simulink model "SIL_swarm_Vasarhelyi"  (R2020b)
settings: Solver=FixedStepAuto  StartTime=0.0  StopTime=T  FixedStep=sim_rate  RelTol=1e-3  EnableMultiTasking=on
model workspace (MAT data in the model file):
  SL_ROS_VariableLengthArrays_MaxSizes : object (value not decoded)
undefined symbols (not defined in the file): airspeed_ref, Altitude_ref, DiscIntNeverNeededParam, Elevators, N_Waypoints, p_swarm, Propeller, Radius_waypoint, RightAileron, RightFlap, Rudder, Waypoints
libraries: robotlib x21, simulink x10, eeGeneralControl x5, dspvision x5
(part 2 of 4)

== system SIL_swarm_Vasarhelyi/Cessna 4/Controle de Direção ==
  Yaw : Inport
  X : Inport  Port=2
  Y : Inport  Port=3
  Y Ref : Inport  Port=4
  X Ref : Inport  Port=5
  Atan2 : Trigonometry  Operator=atan2
  Discrete Derivative : simulink/Discrete/Discrete Derivative  gainval=1.0  ICPrevScaledInput=0.0  OutMin=[]  OutMax=[]  OutDataType=fixdt(1, 16)  OutScaling=2^-10  DoSatur=off
  Discrete-Time Integrator : DiscreteIntegrator  SampleTime=-1  ICPrevOutput=DiscIntNeverNeededParam  ICPrevScaledInput=DiscIntNeverNeededParam
  Kd : Gain  Gain=3.0
  Ki : Gain  Gain=0.0
  Kp : Gain  Gain=1.6616
  Mux1 : Mux  Inputs=2
  Mux2 : Mux  Inputs=2
  Mux3 : Mux  Inputs=2
  Saturation : Saturate  UpperLimit=0.226893  LowerLimit=-0.226893
  Sum2 : Sum  Inputs=|+-
  Sum3 : Sum  Inputs=|+-
  Sum4 : Sum  Inputs=|+-
  Sum5 : Sum  Inputs=+++
  neg : Gain  Gain=-1
  yaw_error : Outport
  Roll Ref : Outport  Port=2
  guidance_error : Outport  Port=3
  wires:
  Mux1/1 -> Mux3/1
  Mux2/1 -> Mux3/2
  Saturation/1 -> neg/1
  neg/1 -> Roll Ref/1
  Sum3/1 -> Atan2/1
  Y/1 -> Sum3/2, Mux2/2
  Y Ref/1 -> Sum3/1, Mux2/1
  X Ref/1 -> Sum2/1, Mux1/1
  X/1 -> Sum2/2, Mux1/2
  Sum2/1 -> Atan2/2
  Atan2/1 -> Sum4/1
  Yaw/1 -> Sum4/2
  Mux3/1 -> guidance_error/1
  Sum5/1 -> Saturation/1
  Kp/1 -> Sum5/2
  Kd/1 -> Sum5/1
  Discrete Derivative/1 -> Kd/1
  Discrete-Time Integrator/1 -> Ki/1
  Sum4/1 -> Discrete-Time Integrator/1, Kp/1, Discrete Derivative/1, yaw_error/1
  Ki/1 -> Sum5/3

== system SIL_swarm_Vasarhelyi/Cessna 4/High-Level ==
  Pos : Inport
  Altitude ref : Inport  Port=2
  Xi : Inport  Port=3
  Bus Selector2 : BusSelector  OutputSignals=X,Y,Altitude
  Filtered Derivative Discrete : eeGeneralControl/Filtered Derivative (Discrete or Continuous)  K=1  T=0.001  B=inf  A=-inf  minRatio=10  init_option=Inherited from block input  x0=0  Ts=-1
      settings: SourceProductBaseCode=PS
  Gerador de Waypoints : Subsystem
  Mux : Mux  Inputs=3
  Mux1 : Mux  Inputs=3
  Terminator2 : Terminator
  Vasarhelyi Algorithm : Subsystem
  Velocity Direction : MATLAB Function  TreatAsAtomicUnit=on
  Y Ref : Outport
  X Ref : Outport  Port=2
  vel : Outport  Port=3
  u_ref : Outport  Port=4
  Waypoints : Outport  Port=5
  wires:
  Mux1/1 -> Waypoints/1, Velocity Direction/2(wp)
  Velocity Direction/1(u_ref) -> u_ref/1, Vasarhelyi Algorithm/3(u_ref)
  Pos/1 -> Bus Selector2/1
  Altitude ref/1 -> Mux1/3
  Gerador de Waypoints/2(Y Ref) -> Mux1/2
  Gerador de Waypoints/1(X Ref) -> Mux1/1
  Bus Selector2/1 -> Mux/1  "<X>"
  Bus Selector2/2 -> Mux/2  "<Y>"
  Bus Selector2/3 -> Mux/3  "<Altitude>"
  Mux/1 -> Filtered Derivative Discrete/1, Vasarhelyi Algorithm/1(pos_i), Velocity Direction/1(pos)
  Filtered Derivative Discrete/1 -> vel/1
  Xi/1 -> Vasarhelyi Algorithm/2(pqj)
  Vasarhelyi Algorithm/1(X) -> X Ref/1
  Vasarhelyi Algorithm/2(Y) -> Y Ref/1
  Vasarhelyi Algorithm/3(Z) -> Terminator2/1
  Vasarhelyi Algorithm/4(Xi) -> Gerador de Waypoints/1(Xi)

== system SIL_swarm_Vasarhelyi/Cessna 4/ROS Communication ==
  Profundor : Inport
  Rudder : Inport  Port=2
  Aileron : Inport  Port=3
  Throttle : Inport  Port=4
  Constant : Constant  Value=0
  Constant1 : Constant  Value=0
  Envio e Recepção de Dados do ROS : Subsystem
  Terminator2 : Terminator
  Roll : Outport
  Pitch : Outport  Port=2
  Yaw : Outport  Port=3
  ECEF Y : Outport  Port=4
  ECEF X : Outport  Port=5
  ECEF Z : Outport  Port=6
  Velocity : Outport  Port=7
  Xi : Outport  Port=8
  wires:
  Profundor/1 -> Envio e Recepção de Dados do ROS/2(Elevators)
  Constant/1 -> Envio e Recepção de Dados do ROS/3(Flap)
  Aileron/1 -> Envio e Recepção de Dados do ROS/4(Aileron)
  Envio e Recepção de Dados do ROS/1(Pitch) -> Pitch/1
  Envio e Recepção de Dados do ROS/4(ECEF X) -> ECEF X/1
  Envio e Recepção de Dados do ROS/5(ECEF Y) -> ECEF Y/1
  Envio e Recepção de Dados do ROS/2(Yaw) -> Yaw/1
  Envio e Recepção de Dados do ROS/3(Roll) -> Roll/1
  Envio e Recepção de Dados do ROS/6(ECEF Z) -> ECEF Z/1
  Envio e Recepção de Dados do ROS/7(Velocity) -> Velocity/1
  Rudder/1 -> Terminator2/1
  Envio e Recepção de Dados do ROS/8(Xi) -> Xi/1
  Throttle/1 -> Envio e Recepção de Dados do ROS/5(Propeller)
  Constant1/1 -> Envio e Recepção de Dados do ROS/1(Rudder)

== system SIL_swarm_Vasarhelyi/Cessna 5/Attitude Control ==
  note: bota po
  Vel ref : Inport
  Euler Angles : Inport  Port=2
  Roll_ref : Inport  Port=3
  Altitude : Inport  Port=4
  Vel_in : Inport  Port=5
  Altitude ref : Inport  Port=6
  Bus Selector : BusSelector  OutputSignals=Pitch,Roll,Yaw
  Constant : Constant  Value=0
  Controle de Altitude : Subsystem
  Controle de Velocidade : Subsystem
  Gain : Gain  Gain=-1
  Servo : Subsystem
  Sum1 : Sum  Inputs=|+-
  Sum3 : Sum  Inputs=+-|
  Sum5 : Sum  Inputs=+-|
  Z Take-off Ref : Constant  Value=5
  Profundor : Outport
  Rudder : Outport  Port=2
  Aileron : Outport  Port=3
  Throtlle : Outport  Port=4
  altitude_e : Outport  Port=5
  velocity_e : Outport  Port=6
  roll_e : Outport  Port=7
  wires:
  Roll_ref/1 -> Sum1/1  "Roll Ref"
  Constant/1 -> Sum5/1  "Yaw Ref"
  Servo/4(Throtlle) -> Throtlle/1
  Servo/2(Aileron) -> Aileron/1
  Servo/3(Rudder) -> Rudder/1
  Servo/1(Profundor) -> Profundor/1
  Z Take-off Ref/1 -> Servo/6(Altitude Ref)
  Altitude/1 -> Controle de Altitude/2(Altitude), Servo/5(Altitude)
  Gain/1 -> Sum3/2
  Sum5/1 -> Servo/3(Yaw Attitude)
  Bus Selector/3 -> Sum5/2  "<Yaw>"
  Sum3/1 -> Servo/1(Pitch Attitude)
  Euler Angles/1 -> Bus Selector/1
  Bus Selector/1 -> Gain/1  "<Pitch>"
  Bus Selector/2 -> Sum1/2  "<Roll>"
  Controle de Velocidade/1(Propeller Target) -> Servo/4(Vel_in)
  Controle de Altitude/1(Pitch_ref) -> Sum3/1
  Vel ref/1 -> Controle de Velocidade/1(Velocity Ref)
  Altitude ref/1 -> Controle de Altitude/1(Altitude Ref)
  Sum1/1 -> roll_e/1, Servo/2(Roll Attitude)
  Vel_in/1 -> Controle de Velocidade/2(Velocity)
  Controle de Altitude/2(altitude_error) -> altitude_e/1
  Controle de Velocidade/2(velocity_error) -> velocity_e/1

== system SIL_swarm_Vasarhelyi/Cessna 5/Controle de Direção ==
  Yaw : Inport
  X : Inport  Port=2
  Y : Inport  Port=3
  Y Ref : Inport  Port=4
  X Ref : Inport  Port=5
  Atan2 : Trigonometry  Operator=atan2
  Discrete Derivative : simulink/Discrete/Discrete Derivative  gainval=1.0  ICPrevScaledInput=0.0  OutMin=[]  OutMax=[]  OutDataType=fixdt(1, 16)  OutScaling=2^-10  DoSatur=off
  Discrete-Time Integrator : DiscreteIntegrator  SampleTime=-1  ICPrevOutput=DiscIntNeverNeededParam  ICPrevScaledInput=DiscIntNeverNeededParam
  Kd : Gain  Gain=3.0
  Ki : Gain  Gain=0.0
  Kp : Gain  Gain=1.6616
  Mux1 : Mux  Inputs=2
  Mux2 : Mux  Inputs=2
  Mux3 : Mux  Inputs=2
  Saturation : Saturate  UpperLimit=0.226893  LowerLimit=-0.226893
  Sum2 : Sum  Inputs=|+-
  Sum3 : Sum  Inputs=|+-
  Sum4 : Sum  Inputs=|+-
  Sum5 : Sum  Inputs=+++
  neg : Gain  Gain=-1
  yaw_error : Outport
  Roll Ref : Outport  Port=2
  guidance_error : Outport  Port=3
  wires:
  Mux1/1 -> Mux3/1
  Mux2/1 -> Mux3/2
  Saturation/1 -> neg/1
  neg/1 -> Roll Ref/1
  Sum3/1 -> Atan2/1
  Y/1 -> Sum3/2, Mux2/2
  Y Ref/1 -> Sum3/1, Mux2/1
  X Ref/1 -> Sum2/1, Mux1/1
  X/1 -> Sum2/2, Mux1/2
  Sum2/1 -> Atan2/2
  Atan2/1 -> Sum4/1
  Yaw/1 -> Sum4/2
  Mux3/1 -> guidance_error/1
  Sum5/1 -> Saturation/1
  Kp/1 -> Sum5/2
  Kd/1 -> Sum5/1
  Discrete Derivative/1 -> Kd/1
  Discrete-Time Integrator/1 -> Ki/1
  Sum4/1 -> Discrete-Time Integrator/1, Kp/1, Discrete Derivative/1, yaw_error/1
  Ki/1 -> Sum5/3

== system SIL_swarm_Vasarhelyi/Cessna 5/High-Level ==
  Pos : Inport
  Altitude ref : Inport  Port=2
  Xi : Inport  Port=3
  Bus Selector2 : BusSelector  OutputSignals=X,Y,Altitude
  Filtered Derivative Discrete : eeGeneralControl/Filtered Derivative (Discrete or Continuous)  K=1  T=0.001  B=inf  A=-inf  minRatio=10  init_option=Inherited from block input  x0=0  Ts=-1
      settings: SourceProductBaseCode=PS
  Gerador de Waypoints : Subsystem
  Mux : Mux  Inputs=3
  Mux1 : Mux  Inputs=3
  Terminator2 : Terminator
  Vasarhelyi Algorithm : Subsystem
  Velocity Direction : MATLAB Function  TreatAsAtomicUnit=on
  Y Ref : Outport
  X Ref : Outport  Port=2
  vel : Outport  Port=3
  u_ref : Outport  Port=4
  Waypoints : Outport  Port=5
  wires:
  Mux1/1 -> Waypoints/1, Velocity Direction/2(wp)
  Velocity Direction/1(u_ref) -> u_ref/1, Vasarhelyi Algorithm/3(u_ref)
  Pos/1 -> Bus Selector2/1
  Altitude ref/1 -> Mux1/3
  Gerador de Waypoints/2(Y Ref) -> Mux1/2
  Gerador de Waypoints/1(X Ref) -> Mux1/1
  Bus Selector2/1 -> Mux/1  "<X>"
  Bus Selector2/2 -> Mux/2  "<Y>"
  Bus Selector2/3 -> Mux/3  "<Altitude>"
  Mux/1 -> Filtered Derivative Discrete/1, Vasarhelyi Algorithm/1(pos_i), Velocity Direction/1(pos)
  Filtered Derivative Discrete/1 -> vel/1
  Xi/1 -> Vasarhelyi Algorithm/2(pqj)
  Vasarhelyi Algorithm/1(X) -> X Ref/1
  Vasarhelyi Algorithm/2(Y) -> Y Ref/1
  Vasarhelyi Algorithm/3(Z) -> Terminator2/1
  Vasarhelyi Algorithm/4(Xi) -> Gerador de Waypoints/1(Xi)

== system SIL_swarm_Vasarhelyi/Cessna 5/ROS Communication ==
  Profundor : Inport
  Rudder : Inport  Port=2
  Aileron : Inport  Port=3
  Throttle : Inport  Port=4
  Constant : Constant  Value=0
  Constant1 : Constant  Value=0
  Envio e Recepção de Dados do ROS : Subsystem
  Terminator2 : Terminator
  Roll : Outport
  Pitch : Outport  Port=2
  Yaw : Outport  Port=3
  ECEF Y : Outport  Port=4
  ECEF X : Outport  Port=5
  ECEF Z : Outport  Port=6
  Velocity : Outport  Port=7
  Xi : Outport  Port=8
  wires:
  Profundor/1 -> Envio e Recepção de Dados do ROS/2(Elevators)
  Constant/1 -> Envio e Recepção de Dados do ROS/3(Flap)
  Aileron/1 -> Envio e Recepção de Dados do ROS/4(Aileron)
  Envio e Recepção de Dados do ROS/1(Pitch) -> Pitch/1
  Envio e Recepção de Dados do ROS/4(ECEF X) -> ECEF X/1
  Envio e Recepção de Dados do ROS/5(ECEF Y) -> ECEF Y/1
  Envio e Recepção de Dados do ROS/2(Yaw) -> Yaw/1
  Envio e Recepção de Dados do ROS/3(Roll) -> Roll/1
  Envio e Recepção de Dados do ROS/6(ECEF Z) -> ECEF Z/1
  Envio e Recepção de Dados do ROS/7(Velocity) -> Velocity/1
  Rudder/1 -> Terminator2/1
  Envio e Recepção de Dados do ROS/8(Xi) -> Xi/1
  Throttle/1 -> Envio e Recepção de Dados do ROS/5(Propeller)
  Constant1/1 -> Envio e Recepção de Dados do ROS/1(Rudder)

== system SIL_swarm_Vasarhelyi/Cessna 1/Attitude Control/Controle de Altitude ==
  Altitude Ref : Inport
  Altitude : Inport  Port=2
  Derivative1 : Derivative
  Kd : Gain  Gain=0.00162
  Kp : Gain  Gain=0.1
  Saturation : Saturate  UpperLimit=0.785398  LowerLimit=-0.785398
  Sum : Sum  Inputs=|+-
  Sum5 : Sum  Inputs=++|
  Pitch_ref : Outport
  altitude_error : Outport  Port=2
  wires:
  Saturation/1 -> Pitch_ref/1
  Altitude Ref/1 -> Sum/1
  Altitude/1 -> Sum/2
  Kp/1 -> Sum5/2
  Kd/1 -> Sum5/1
  Derivative1/1 -> Kd/1
  Sum5/1 -> Saturation/1
  Sum/1 -> Derivative1/1, Kp/1, altitude_error/1

== system SIL_swarm_Vasarhelyi/Cessna 1/Attitude Control/Controle de Velocidade ==
  Velocity Ref : Inport
  Velocity : Inport  Port=2
  K_prop : Gain  Gain=0.08
  PID Velocidade : Subsystem
  Propeller Ref : Constant  Value=0.7
  Saturation3 : Saturate  UpperLimit=0.8  LowerLimit=0.6
  Sum1 : Sum  Inputs=+|+
  Sum7 : Sum  Inputs=+|-
  Target Propeller : Scope
  Velocity Error : Scope
  Propeller Target : Outport
  velocity_error : Outport  Port=2
  wires:
  Velocity/1 -> Sum7/2
  Velocity Ref/1 -> Sum7/1
  PID Velocidade/1(ev) -> K_prop/1
  Saturation3/1 -> Target Propeller/1, Propeller Target/1
  Propeller Ref/1 -> Sum1/2
  K_prop/1 -> Sum1/1
  Sum1/1 -> Saturation3/1
  Sum7/1 -> PID Velocidade/1(e_vel), velocity_error/1, Velocity Error/1

== system SIL_swarm_Vasarhelyi/Cessna 1/Attitude Control/Servo ==
  Pitch Attitude : Inport
  Roll Attitude : Inport  Port=2
  Yaw Attitude : Inport  Port=3
  Vel_in : Inport  Port=4
  Altitude : Inport  Port=5
  Altitude Ref : Inport  Port=6
  Gain1 : Gain  Gain=-1
  Gain2 : Gain
  Gain3 : Gain
  GreaterThanOrEqual : RelationalOperator  OutDataTypeStr=boolean  RndMeth=Simplest
  Saturation2 : Saturate  UpperLimit=0.0523599  LowerLimit=-0.0523599
  Saturation4 : Saturate  UpperLimit=0.0523599  LowerLimit=-0.0523599
  Saturation6 : Saturate  UpperLimit=0.0872665  LowerLimit=-0.0872665
  Switch{,1..3} (4 alike) : Switch  Criteria=u2 ~= 0
  Take-Off : Subsystem
  Profundor : Outport
  Aileron : Outport  Port=2
  Rudder : Outport  Port=3
  Throtlle : Outport  Port=4
  wires:
  GreaterThanOrEqual/1 -> Switch3/2, Switch2/2, Switch1/2, Switch/2
  Altitude Ref/1 -> GreaterThanOrEqual/2
  Take-Off/3(Rudder) -> Switch3/3
  Take-Off/2(Aileron) -> Switch2/3
  Altitude/1 -> GreaterThanOrEqual/1
  Switch3/1 -> Rudder/1
  Vel_in/1 -> Switch/1
  Switch/1 -> Throtlle/1
  Take-Off/4(Propeller) -> Switch/3
  Switch1/1 -> Profundor/1
  Take-Off/1(Elevators) -> Switch1/3
  Switch2/1 -> Aileron/1
  Saturation2/1 -> Switch2/1
  Saturation4/1 -> Switch1/1
  Saturation6/1 -> Switch3/1
  Gain1/1 -> Saturation6/1
  Yaw Attitude/1 -> Gain1/1
  Roll Attitude/1 -> Gain3/1
  Pitch Attitude/1 -> Gain2/1
  Gain2/1 -> Saturation4/1
  Gain3/1 -> Saturation2/1

== system SIL_swarm_Vasarhelyi/Cessna 1/High-Level/Gerador de Waypoints ==
  Xi : Inport
  Constant : Constant  Value=Radius_waypoint
  Constant1 : Constant  Value=Waypoints
  Constant2 : Constant  Value=N_Waypoints
  Constant3 : Constant  Value=p_swarm.r
  Display : Display
  Memory : Memory
  Next Waypoint : MATLAB Function  TreatAsAtomicUnit=on
  X Ref : Outport
  Y Ref : Outport  Port=2
  wires:
  Memory/1 -> Next Waypoint/6("Current_Waypoint ")
  Constant1/1 -> Next Waypoint/4(Waypoints)
  Xi/1 -> Next Waypoint/1(Xi)
  Constant3/1 -> Next Waypoint/3(p_swarm_r)
  Constant2/1 -> Next Waypoint/5(N_Waypoints)
  Next Waypoint/3(Current_Waypoint) -> Display/1, Memory/1
  Constant/1 -> Next Waypoint/2(R)
  Next Waypoint/1(X_ref) -> X Ref/1
  Next Waypoint/2(Y_ref) -> Y Ref/1

== system SIL_swarm_Vasarhelyi/Cessna 1/High-Level/Vasarhelyi Algorithm ==
  pos_i : Inport
  pqj : Inport  Port=2
  u_ref : Inport  Port=3
  Agents Number : Constant  Value=5
  Demux : Demux  Outputs=3
  Discrete Derivative : simulink/Discrete/Discrete Derivative  gainval=1.0  ICPrevScaledInput=0.0  OutMin=[]  OutMax=[]  OutDataType=fixdt(1, 16)  OutScaling=2^-10  DoSatur=off
  Discrete-Time Integrator : DiscreteIntegrator  SampleTime=-1  ICPrevOutput=DiscIntNeverNeededParam  ICPrevScaledInput=DiscIntNeverNeededParam
  Parameters : Subsystem
  Vasarhelyi Algorithm : MATLAB Function  TreatAsAtomicUnit=on
  dt : Constant  Value=0.01
  pos and vel of uavs : MATLAB Function  TreatAsAtomicUnit=on
  r_agent : Constant  Value=p_swarm.r_agent
  X : Outport
  Y : Outport  Port=2
  Z : Outport  Port=3
  Xi : Outport  Port=4
  wires:
  Agents Number/1 -> pos and vel of uavs/1(nb_agents)
  u_ref/1 -> Vasarhelyi Algorithm/4(u_ref)
  Vasarhelyi Algorithm/1(vel_command) -> Discrete-Time Integrator/1
  dt/1 -> Vasarhelyi Algorithm/5(dt)
  pqj/1 -> pos and vel of uavs/3(pqj)
  r_agent/1 -> Vasarhelyi Algorithm/6(r_agent)
  Discrete-Time Integrator/1 -> Demux/1
  pos and vel of uavs/1(pos) -> Discrete Derivative/1, Vasarhelyi Algorithm/2(pos), Xi/1
  Demux/2 -> Y/1
  pos_i/1 -> pos and vel of uavs/2(pos_i)
  Demux/1 -> X/1
  Demux/3 -> Z/1
  Discrete Derivative/1 -> Vasarhelyi Algorithm/3(vel)
  Parameters/1(p_swarm) -> Vasarhelyi Algorithm/1(p_swarm_par)

== system SIL_swarm_Vasarhelyi/Cessna 1/ROS Communication/Envio e Recepção de Dados do ROS ==
  note: ROS Receive
  Rudder : Inport
  Elevators : Inport  Port=2
  Flap : Inport  Port=3
  Aileron : Inport  Port=4
  Propeller : Inport  Port=5
  Blank Message : robotlib/Blank Message  messageClass=Message  entityType=aircraft_messages/Control_Surfaces  messageType=aircraft_messages/Control_Surfaces  SampleTime=-1  legacyBusStruct=off
  Bus Assignment1 : BusAssignment  AssignedSignals=Rudder,Elevators,RightFlap,RightAileron,Propeller
  Bus Selector1 : BusSelector  OutputSignals=Roll,Pitch,Yaw,PositionX,PositionY,PositionZ,Velocity
  Odometry : robotlib/Subscribe  topicSource=Select from ROS network  topic=/uav1/ground_truth/Odometry  messageType=aircraft_communication/Odom  SampleTime=-1  legacyBusStruct=off  messageQueueLength=1
  Publish : robotlib/Publish  topicSource=Select from ROS network  topic=/uav1/command  messageType=aircraft_messages/Control_Surfaces  legacyBusStruct=off  messageQueueLength=1
  Subscribe Odometry : Subsystem  TreatAsAtomicUnit=on
  Terminator1 : Terminator
  Terminator2 : Terminator
  Wifi Data : robotlib/Subscribe  topicSource=Select from ROS network  topic=/uav1/Communication  messageType=aircraft_communication/NetworkComm  SampleTime=-1  legacyBusStruct=off  messageQueueLength=1
  Pitch : Outport
  Yaw : Outport  Port=2
  Roll : Outport  Port=3
  ECEF X : Outport  Port=4
  ECEF Y : Outport  Port=5
  ECEF Z : Outport  Port=6
  Velocity : Outport  Port=7
  Xi : Outport  Port=8
  wires:
  Subscribe Odometry/5(ECEF Y) -> ECEF Y/1
  Subscribe Odometry/4(ECEF X) -> ECEF X/1
  Subscribe Odometry/2(Pitch) -> Pitch/1
  Subscribe Odometry/6(ECEF Z) -> ECEF Z/1
  Subscribe Odometry/8(Xi) -> Xi/1
  Subscribe Odometry/7(Velocity Out) -> Velocity/1
  Odometry/2 -> Bus Selector1/1
  Bus Selector1/4 -> Subscribe Odometry/4(ECEF_X)  "<PositionX>"
  Bus Selector1/5 -> Subscribe Odometry/5(ECEF_Y)  "<PositionY>"
  Bus Selector1/6 -> Subscribe Odometry/6(ECEF_Z)  "<PositionZ>"
  Wifi Data/2 -> Subscribe Odometry/8(Communication)
  Bus Selector1/7 -> Subscribe Odometry/7(Vel)  "<Velocity>"
  Bus Selector1/2 -> Subscribe Odometry/2(Pitch in)  "<Pitch>"
  Bus Selector1/1 -> Subscribe Odometry/1(Roll in)  "<Roll>"
  Bus Selector1/3 -> Subscribe Odometry/3(Yaw in)  "<Yaw>"
  Subscribe Odometry/3(Yaw) -> Yaw/1
  Subscribe Odometry/1(Roll) -> Roll/1
  Wifi Data/1 -> Terminator2/1
  Aileron/1 -> Bus Assignment1/5
  Blank Message/1 -> Bus Assignment1/1
  Flap/1 -> Bus Assignment1/4
  Elevators/1 -> Bus Assignment1/3
  Rudder/1 -> Bus Assignment1/2
  Bus Assignment1/1 -> Publish/1
  Propeller/1 -> Bus Assignment1/6
  Odometry/1 -> Terminator1/1

== system SIL_swarm_Vasarhelyi/Cessna 2/Attitude Control/Controle de Altitude ==
  Altitude Ref : Inport
  Altitude : Inport  Port=2
  Derivative1 : Derivative
  Kd : Gain  Gain=0.00162
  Kp : Gain  Gain=0.1
  Saturation : Saturate  UpperLimit=0.785398  LowerLimit=-0.785398
  Sum : Sum  Inputs=|+-
  Sum5 : Sum  Inputs=++|
  Pitch_ref : Outport
  altitude_error : Outport  Port=2
  wires:
  Saturation/1 -> Pitch_ref/1
  Altitude Ref/1 -> Sum/1
  Altitude/1 -> Sum/2
  Kp/1 -> Sum5/2
  Kd/1 -> Sum5/1
  Derivative1/1 -> Kd/1
  Sum5/1 -> Saturation/1
  Sum/1 -> Derivative1/1, Kp/1, altitude_error/1

== system SIL_swarm_Vasarhelyi/Cessna 2/Attitude Control/Controle de Velocidade ==
  Velocity Ref : Inport
  Velocity : Inport  Port=2
  K_prop : Gain  Gain=0.08
  PID Velocidade : Subsystem
  Propeller Ref : Constant  Value=0.7
  Saturation3 : Saturate  UpperLimit=0.8  LowerLimit=0.6
  Sum1 : Sum  Inputs=+|+
  Sum7 : Sum  Inputs=+|-
  Target Propeller : Scope
  Velocity Error : Scope
  Propeller Target : Outport
  velocity_error : Outport  Port=2
  wires:
  Velocity/1 -> Sum7/2
  Velocity Ref/1 -> Sum7/1
  PID Velocidade/1(ev) -> K_prop/1
  Saturation3/1 -> Target Propeller/1, Propeller Target/1
  Propeller Ref/1 -> Sum1/2
  K_prop/1 -> Sum1/1
  Sum1/1 -> Saturation3/1
  Sum7/1 -> PID Velocidade/1(e_vel), velocity_error/1, Velocity Error/1

== system SIL_swarm_Vasarhelyi/Cessna 2/Attitude Control/Servo ==
  Pitch Attitude : Inport
  Roll Attitude : Inport  Port=2
  Yaw Attitude : Inport  Port=3
  Vel_in : Inport  Port=4
  Altitude : Inport  Port=5
  Altitude Ref : Inport  Port=6
  Gain1 : Gain  Gain=-1
  Gain2 : Gain
  Gain3 : Gain
  GreaterThanOrEqual : RelationalOperator  OutDataTypeStr=boolean  RndMeth=Simplest
  Saturation2 : Saturate  UpperLimit=0.0523599  LowerLimit=-0.0523599
  Saturation4 : Saturate  UpperLimit=0.0523599  LowerLimit=-0.0523599
  Saturation6 : Saturate  UpperLimit=0.0872665  LowerLimit=-0.0872665
  Switch{,1..3} (4 alike) : Switch  Criteria=u2 ~= 0
  Take-Off : Subsystem
  Profundor : Outport
  Aileron : Outport  Port=2
  Rudder : Outport  Port=3
  Throtlle : Outport  Port=4
  wires:
  GreaterThanOrEqual/1 -> Switch3/2, Switch2/2, Switch1/2, Switch/2
  Altitude Ref/1 -> GreaterThanOrEqual/2
  Take-Off/3(Rudder) -> Switch3/3
  Take-Off/2(Aileron) -> Switch2/3
  Altitude/1 -> GreaterThanOrEqual/1
  Switch3/1 -> Rudder/1
  Vel_in/1 -> Switch/1
  Switch/1 -> Throtlle/1
  Take-Off/4(Propeller) -> Switch/3
  Switch1/1 -> Profundor/1
  Take-Off/1(Elevators) -> Switch1/3
  Switch2/1 -> Aileron/1
  Saturation2/1 -> Switch2/1
  Saturation4/1 -> Switch1/1
  Saturation6/1 -> Switch3/1
  Gain1/1 -> Saturation6/1
  Yaw Attitude/1 -> Gain1/1
  Roll Attitude/1 -> Gain3/1
  Pitch Attitude/1 -> Gain2/1
  Gain2/1 -> Saturation4/1
  Gain3/1 -> Saturation2/1

== system SIL_swarm_Vasarhelyi/Cessna 2/High-Level/Gerador de Waypoints ==
  Xi : Inport
  Constant : Constant  Value=Radius_waypoint
  Constant1 : Constant  Value=Waypoints
  Constant2 : Constant  Value=N_Waypoints
  Constant3 : Constant  Value=p_swarm.r
  Display : Display
  Memory : Memory
  Next Waypoint : MATLAB Function  TreatAsAtomicUnit=on
  X Ref : Outport
  Y Ref : Outport  Port=2
  wires:
  Memory/1 -> Next Waypoint/6("Current_Waypoint ")
  Constant1/1 -> Next Waypoint/4(Waypoints)
  Xi/1 -> Next Waypoint/1(Xi)
  Constant3/1 -> Next Waypoint/3(p_swarm_r)
  Constant2/1 -> Next Waypoint/5(N_Waypoints)
  Next Waypoint/3(Current_Waypoint) -> Display/1, Memory/1
  Constant/1 -> Next Waypoint/2(R)
  Next Waypoint/1(X_ref) -> X Ref/1
  Next Waypoint/2(Y_ref) -> Y Ref/1

== system SIL_swarm_Vasarhelyi/Cessna 2/High-Level/Vasarhelyi Algorithm ==
  pos_i : Inport
  pqj : Inport  Port=2
  u_ref : Inport  Port=3
  Agents Number : Constant  Value=5
  Demux : Demux  Outputs=3
  Discrete Derivative : simulink/Discrete/Discrete Derivative  gainval=1.0  ICPrevScaledInput=0.0  OutMin=[]  OutMax=[]  OutDataType=fixdt(1, 16)  OutScaling=2^-10  DoSatur=off
  Discrete-Time Integrator : DiscreteIntegrator  SampleTime=-1  ICPrevOutput=DiscIntNeverNeededParam  ICPrevScaledInput=DiscIntNeverNeededParam
  Parameters : Subsystem
  Vasarhelyi Algorithm : MATLAB Function  TreatAsAtomicUnit=on
  dt : Constant  Value=0.01
  pos and vel of uavs : MATLAB Function  TreatAsAtomicUnit=on
  r_agent : Constant  Value=p_swarm.r_agent
  X : Outport
  Y : Outport  Port=2
  Z : Outport  Port=3
  Xi : Outport  Port=4
  wires:
  Agents Number/1 -> pos and vel of uavs/1(nb_agents)
  u_ref/1 -> Vasarhelyi Algorithm/4(u_ref)
  Vasarhelyi Algorithm/1(vel_command) -> Discrete-Time Integrator/1
  dt/1 -> Vasarhelyi Algorithm/5(dt)
  pqj/1 -> pos and vel of uavs/3(pqj)
  r_agent/1 -> Vasarhelyi Algorithm/6(r_agent)
  Discrete-Time Integrator/1 -> Demux/1
  pos and vel of uavs/1(pos) -> Discrete Derivative/1, Vasarhelyi Algorithm/2(pos), Xi/1
  Demux/2 -> Y/1
  pos_i/1 -> pos and vel of uavs/2(pos_i)
  Demux/1 -> X/1
  Demux/3 -> Z/1
  Discrete Derivative/1 -> Vasarhelyi Algorithm/3(vel)
  Parameters/1(p_swarm) -> Vasarhelyi Algorithm/1(p_swarm_par)

== system SIL_swarm_Vasarhelyi/Cessna 2/ROS Communication/Envio e Recepção de Dados do ROS ==
  note: ROS Receive
  Rudder : Inport
  Elevators : Inport  Port=2
  Flap : Inport  Port=3
  Aileron : Inport  Port=4
  Propeller : Inport  Port=5
  Blank Message : robotlib/Blank Message  messageClass=Message  entityType=aircraft_messages/Control_Surfaces  messageType=aircraft_messages/Control_Surfaces  SampleTime=-1  legacyBusStruct=off
  Bus Assignment1 : BusAssignment  AssignedSignals=Rudder,Elevators,RightFlap,RightAileron,Propeller
  Bus Selector1 : BusSelector  OutputSignals=Roll,Pitch,Yaw,PositionX,PositionY,PositionZ,Velocity
  Odometry : robotlib/Subscribe  topicSource=Select from ROS network  topic=/uav2/ground_truth/Odometry  messageType=aircraft_communication/Odom  SampleTime=-1  legacyBusStruct=off  messageQueueLength=1
  Publish : robotlib/Publish  topicSource=Select from ROS network  topic=/uav2/command  messageType=aircraft_messages/Control_Surfaces  legacyBusStruct=off  messageQueueLength=1
  Subscribe Odometry : Subsystem  TreatAsAtomicUnit=on
  Terminator1 : Terminator
  Terminator2 : Terminator
  Wifi Data : robotlib/Subscribe  topicSource=Select from ROS network  topic=/uav2/Communication  messageType=aircraft_communication/NetworkComm  SampleTime=-1  legacyBusStruct=off  messageQueueLength=1
  Pitch : Outport
  Yaw : Outport  Port=2
  Roll : Outport  Port=3
  ECEF X : Outport  Port=4
  ECEF Y : Outport  Port=5
  ECEF Z : Outport  Port=6
  Velocity : Outport  Port=7
  Xi : Outport  Port=8
  wires:
  Subscribe Odometry/5(ECEF Y) -> ECEF Y/1
  Subscribe Odometry/4(ECEF X) -> ECEF X/1
  Subscribe Odometry/2(Pitch) -> Pitch/1
  Subscribe Odometry/6(ECEF Z) -> ECEF Z/1
  Subscribe Odometry/8(Xi) -> Xi/1
  Subscribe Odometry/7(Velocity Out) -> Velocity/1
  Odometry/2 -> Bus Selector1/1
  Bus Selector1/4 -> Subscribe Odometry/4(ECEF_X)  "<PositionX>"
  Bus Selector1/5 -> Subscribe Odometry/5(ECEF_Y)  "<PositionY>"
  Bus Selector1/6 -> Subscribe Odometry/6(ECEF_Z)  "<PositionZ>"
  Wifi Data/2 -> Subscribe Odometry/8(Communication)
  Bus Selector1/7 -> Subscribe Odometry/7(Vel)  "<Velocity>"
  Bus Selector1/2 -> Subscribe Odometry/2(Pitch in)  "<Pitch>"
  Bus Selector1/1 -> Subscribe Odometry/1(Roll in)  "<Roll>"
  Bus Selector1/3 -> Subscribe Odometry/3(Yaw in)  "<Yaw>"
  Subscribe Odometry/3(Yaw) -> Yaw/1
  Subscribe Odometry/1(Roll) -> Roll/1
  Wifi Data/1 -> Terminator2/1
  Aileron/1 -> Bus Assignment1/5
  Blank Message/1 -> Bus Assignment1/1
  Flap/1 -> Bus Assignment1/4
  Elevators/1 -> Bus Assignment1/3
  Rudder/1 -> Bus Assignment1/2
  Bus Assignment1/1 -> Publish/1
  Propeller/1 -> Bus Assignment1/6
  Odometry/1 -> Terminator1/1

== system SIL_swarm_Vasarhelyi/Cessna 3/Attitude Control/Controle de Altitude ==
  Altitude Ref : Inport
  Altitude : Inport  Port=2
  Derivative1 : Derivative
  Kd : Gain  Gain=0.00162
  Kp : Gain  Gain=0.1
  Saturation : Saturate  UpperLimit=0.785398  LowerLimit=-0.785398
  Sum : Sum  Inputs=|+-
  Sum5 : Sum  Inputs=++|
  Pitch_ref : Outport
  altitude_error : Outport  Port=2
  wires:
  Saturation/1 -> Pitch_ref/1
  Altitude Ref/1 -> Sum/1
  Altitude/1 -> Sum/2
  Kp/1 -> Sum5/2
  Kd/1 -> Sum5/1
  Derivative1/1 -> Kd/1
  Sum5/1 -> Saturation/1
  Sum/1 -> Derivative1/1, Kp/1, altitude_error/1

== system SIL_swarm_Vasarhelyi/Cessna 3/Attitude Control/Controle de Velocidade ==
  Velocity Ref : Inport
  Velocity : Inport  Port=2
  K_prop : Gain  Gain=0.08
  PID Velocidade : Subsystem
  Propeller Ref : Constant  Value=0.7
  Saturation3 : Saturate  UpperLimit=0.8  LowerLimit=0.6
  Sum1 : Sum  Inputs=+|+
  Sum7 : Sum  Inputs=+|-
  Target Propeller : Scope
  Velocity Error : Scope
  Propeller Target : Outport
  velocity_error : Outport  Port=2
  wires:
  Velocity/1 -> Sum7/2
  Velocity Ref/1 -> Sum7/1
  PID Velocidade/1(ev) -> K_prop/1
  Saturation3/1 -> Target Propeller/1, Propeller Target/1
  Propeller Ref/1 -> Sum1/2
  K_prop/1 -> Sum1/1
  Sum1/1 -> Saturation3/1
  Sum7/1 -> PID Velocidade/1(e_vel), velocity_error/1, Velocity Error/1

== system SIL_swarm_Vasarhelyi/Cessna 3/Attitude Control/Servo ==
  Pitch Attitude : Inport
  Roll Attitude : Inport  Port=2
  Yaw Attitude : Inport  Port=3
  Vel_in : Inport  Port=4
  Altitude : Inport  Port=5
  Altitude Ref : Inport  Port=6
  Gain1 : Gain  Gain=-1
  Gain2 : Gain
  Gain3 : Gain
  GreaterThanOrEqual : RelationalOperator  OutDataTypeStr=boolean  RndMeth=Simplest
  Saturation2 : Saturate  UpperLimit=0.0523599  LowerLimit=-0.0523599
  Saturation4 : Saturate  UpperLimit=0.0523599  LowerLimit=-0.0523599
  Saturation6 : Saturate  UpperLimit=0.0872665  LowerLimit=-0.0872665
  Switch{,1..3} (4 alike) : Switch  Criteria=u2 ~= 0
  Take-Off : Subsystem
  Profundor : Outport
  Aileron : Outport  Port=2
  Rudder : Outport  Port=3
  Throtlle : Outport  Port=4
  wires:
  GreaterThanOrEqual/1 -> Switch3/2, Switch2/2, Switch1/2, Switch/2
  Altitude Ref/1 -> GreaterThanOrEqual/2
  Take-Off/3(Rudder) -> Switch3/3
  Take-Off/2(Aileron) -> Switch2/3
  Altitude/1 -> GreaterThanOrEqual/1
  Switch3/1 -> Rudder/1
  Vel_in/1 -> Switch/1
  Switch/1 -> Throtlle/1
  Take-Off/4(Propeller) -> Switch/3
  Switch1/1 -> Profundor/1
  Take-Off/1(Elevators) -> Switch1/3
  Switch2/1 -> Aileron/1
  Saturation2/1 -> Switch2/1
  Saturation4/1 -> Switch1/1
  Saturation6/1 -> Switch3/1
  Gain1/1 -> Saturation6/1
  Yaw Attitude/1 -> Gain1/1
  Roll Attitude/1 -> Gain3/1
  Pitch Attitude/1 -> Gain2/1
  Gain2/1 -> Saturation4/1
  Gain3/1 -> Saturation2/1

== system SIL_swarm_Vasarhelyi/Cessna 3/High-Level/Gerador de Waypoints ==
  Xi : Inport
  Constant : Constant  Value=Radius_waypoint
  Constant1 : Constant  Value=Waypoints
  Constant2 : Constant  Value=N_Waypoints
  Constant3 : Constant  Value=p_swarm.r
  Display : Display
  Memory : Memory
  Next Waypoint : MATLAB Function  TreatAsAtomicUnit=on
  X Ref : Outport
  Y Ref : Outport  Port=2
  wires:
  Memory/1 -> Next Waypoint/6("Current_Waypoint ")
  Constant1/1 -> Next Waypoint/4(Waypoints)
  Xi/1 -> Next Waypoint/1(Xi)
  Constant3/1 -> Next Waypoint/3(p_swarm_r)
  Constant2/1 -> Next Waypoint/5(N_Waypoints)
  Next Waypoint/3(Current_Waypoint) -> Display/1, Memory/1
  Constant/1 -> Next Waypoint/2(R)
  Next Waypoint/1(X_ref) -> X Ref/1
  Next Waypoint/2(Y_ref) -> Y Ref/1

== system SIL_swarm_Vasarhelyi/Cessna 3/High-Level/Vasarhelyi Algorithm ==
  pos_i : Inport
  pqj : Inport  Port=2
  u_ref : Inport  Port=3
  Agents Number : Constant  Value=5
  Demux : Demux  Outputs=3
  Discrete Derivative : simulink/Discrete/Discrete Derivative  gainval=1.0  ICPrevScaledInput=0.0  OutMin=[]  OutMax=[]  OutDataType=fixdt(1, 16)  OutScaling=2^-10  DoSatur=off
  Discrete-Time Integrator : DiscreteIntegrator  SampleTime=-1  ICPrevOutput=DiscIntNeverNeededParam  ICPrevScaledInput=DiscIntNeverNeededParam
  Parameters : Subsystem
  Vasarhelyi Algorithm : MATLAB Function  TreatAsAtomicUnit=on
  dt : Constant  Value=0.01
  pos and vel of uavs : MATLAB Function  TreatAsAtomicUnit=on
  r_agent : Constant  Value=p_swarm.r_agent
  X : Outport
  Y : Outport  Port=2
  Z : Outport  Port=3
  Xi : Outport  Port=4
  wires:
  Agents Number/1 -> pos and vel of uavs/1(nb_agents)
  u_ref/1 -> Vasarhelyi Algorithm/4(u_ref)
  Vasarhelyi Algorithm/1(vel_command) -> Discrete-Time Integrator/1
  dt/1 -> Vasarhelyi Algorithm/5(dt)
  pqj/1 -> pos and vel of uavs/3(pqj)
  r_agent/1 -> Vasarhelyi Algorithm/6(r_agent)
  Discrete-Time Integrator/1 -> Demux/1
  pos and vel of uavs/1(pos) -> Discrete Derivative/1, Vasarhelyi Algorithm/2(pos), Xi/1
  Demux/2 -> Y/1
  pos_i/1 -> pos and vel of uavs/2(pos_i)
  Demux/1 -> X/1
  Demux/3 -> Z/1
  Discrete Derivative/1 -> Vasarhelyi Algorithm/3(vel)
  Parameters/1(p_swarm) -> Vasarhelyi Algorithm/1(p_swarm_par)

== system SIL_swarm_Vasarhelyi/Cessna 3/ROS Communication/Envio e Recepção de Dados do ROS ==
  note: ROS Receive
  Rudder : Inport
  Elevators : Inport  Port=2
  Flap : Inport  Port=3
  Aileron : Inport  Port=4
  Propeller : Inport  Port=5
  Blank Message : robotlib/Blank Message  messageClass=Message  entityType=aircraft_messages/Control_Surfaces  messageType=aircraft_messages/Control_Surfaces  SampleTime=-1  legacyBusStruct=off
  Bus Assignment1 : BusAssignment  AssignedSignals=Rudder,Elevators,RightFlap,RightAileron,Propeller
  Bus Selector1 : BusSelector  OutputSignals=Roll,Pitch,Yaw,PositionX,PositionY,PositionZ,Velocity
  Odometry : robotlib/Subscribe  topicSource=Select from ROS network  topic=/uav3/ground_truth/Odometry  messageType=aircraft_communication/Odom  SampleTime=-1  legacyBusStruct=off  messageQueueLength=1
  Publish : robotlib/Publish  topicSource=Select from ROS network  topic=/uav3/command  messageType=aircraft_messages/Control_Surfaces  legacyBusStruct=off  messageQueueLength=1
  Subscribe Odometry : Subsystem  TreatAsAtomicUnit=on
  Terminator1 : Terminator
  Terminator2 : Terminator
  Wifi Data : robotlib/Subscribe  topicSource=Select from ROS network  topic=/uav3/Communication  messageType=aircraft_communication/NetworkComm  SampleTime=-1  legacyBusStruct=off  messageQueueLength=1
  Pitch : Outport
  Yaw : Outport  Port=2
  Roll : Outport  Port=3
  ECEF X : Outport  Port=4
  ECEF Y : Outport  Port=5
  ECEF Z : Outport  Port=6
  Velocity : Outport  Port=7
  Xi : Outport  Port=8
  wires:
  Subscribe Odometry/5(ECEF Y) -> ECEF Y/1
  Subscribe Odometry/4(ECEF X) -> ECEF X/1
  Subscribe Odometry/2(Pitch) -> Pitch/1
  Subscribe Odometry/6(ECEF Z) -> ECEF Z/1
  Subscribe Odometry/8(Xi) -> Xi/1
  Subscribe Odometry/7(Velocity Out) -> Velocity/1
  Odometry/2 -> Bus Selector1/1
  Bus Selector1/4 -> Subscribe Odometry/4(ECEF_X)  "<PositionX>"
  Bus Selector1/5 -> Subscribe Odometry/5(ECEF_Y)  "<PositionY>"
  Bus Selector1/6 -> Subscribe Odometry/6(ECEF_Z)  "<PositionZ>"
  Wifi Data/2 -> Subscribe Odometry/8(Communication)
  Bus Selector1/7 -> Subscribe Odometry/7(Vel)  "<Velocity>"
  Bus Selector1/2 -> Subscribe Odometry/2(Pitch in)  "<Pitch>"
  Bus Selector1/1 -> Subscribe Odometry/1(Roll in)  "<Roll>"
  Bus Selector1/3 -> Subscribe Odometry/3(Yaw in)  "<Yaw>"
  Subscribe Odometry/3(Yaw) -> Yaw/1
  Subscribe Odometry/1(Roll) -> Roll/1
  Wifi Data/1 -> Terminator2/1
  Aileron/1 -> Bus Assignment1/5
  Blank Message/1 -> Bus Assignment1/1
  Flap/1 -> Bus Assignment1/4
  Elevators/1 -> Bus Assignment1/3
  Rudder/1 -> Bus Assignment1/2
  Bus Assignment1/1 -> Publish/1
  Propeller/1 -> Bus Assignment1/6
  Odometry/1 -> Terminator1/1

== system SIL_swarm_Vasarhelyi/Cessna 4/Attitude Control/Controle de Altitude ==
  Altitude Ref : Inport
  Altitude : Inport  Port=2
  Derivative1 : Derivative
  Kd : Gain  Gain=0.00162
  Kp : Gain  Gain=0.1
  Saturation : Saturate  UpperLimit=0.785398  LowerLimit=-0.785398
  Sum : Sum  Inputs=|+-
  Sum5 : Sum  Inputs=++|
  Pitch_ref : Outport
  altitude_error : Outport  Port=2
  wires:
  Saturation/1 -> Pitch_ref/1
  Altitude Ref/1 -> Sum/1
  Altitude/1 -> Sum/2
  Kp/1 -> Sum5/2
  Kd/1 -> Sum5/1
  Derivative1/1 -> Kd/1
  Sum5/1 -> Saturation/1
  Sum/1 -> Derivative1/1, Kp/1, altitude_error/1

== system SIL_swarm_Vasarhelyi/Cessna 4/Attitude Control/Controle de Velocidade ==
  Velocity Ref : Inport
  Velocity : Inport  Port=2
  K_prop : Gain  Gain=0.08
  PID Velocidade : Subsystem
  Propeller Ref : Constant  Value=0.7
  Saturation3 : Saturate  UpperLimit=0.8  LowerLimit=0.6
  Sum1 : Sum  Inputs=+|+
  Sum7 : Sum  Inputs=+|-
  Target Propeller : Scope
  Velocity Error : Scope
  Propeller Target : Outport
  velocity_error : Outport  Port=2
  wires:
  Velocity/1 -> Sum7/2
  Velocity Ref/1 -> Sum7/1
  PID Velocidade/1(ev) -> K_prop/1
  Saturation3/1 -> Target Propeller/1, Propeller Target/1
  Propeller Ref/1 -> Sum1/2
  K_prop/1 -> Sum1/1
  Sum1/1 -> Saturation3/1
  Sum7/1 -> PID Velocidade/1(e_vel), velocity_error/1, Velocity Error/1

== system SIL_swarm_Vasarhelyi/Cessna 4/Attitude Control/Servo ==
  Pitch Attitude : Inport
  Roll Attitude : Inport  Port=2
  Yaw Attitude : Inport  Port=3
  Vel_in : Inport  Port=4
  Altitude : Inport  Port=5
  Altitude Ref : Inport  Port=6
  Gain1 : Gain  Gain=-1
  Gain2 : Gain
  Gain3 : Gain
  GreaterThanOrEqual : RelationalOperator  OutDataTypeStr=boolean  RndMeth=Simplest
  Saturation2 : Saturate  UpperLimit=0.0523599  LowerLimit=-0.0523599
  Saturation4 : Saturate  UpperLimit=0.0523599  LowerLimit=-0.0523599
  Saturation6 : Saturate  UpperLimit=0.0872665  LowerLimit=-0.0872665
  Switch{,1..3} (4 alike) : Switch  Criteria=u2 ~= 0
  Take-Off : Subsystem
  Profundor : Outport
  Aileron : Outport  Port=2
  Rudder : Outport  Port=3
  Throtlle : Outport  Port=4
  wires:
  GreaterThanOrEqual/1 -> Switch3/2, Switch2/2, Switch1/2, Switch/2
  Altitude Ref/1 -> GreaterThanOrEqual/2
  Take-Off/3(Rudder) -> Switch3/3
  Take-Off/2(Aileron) -> Switch2/3
  Altitude/1 -> GreaterThanOrEqual/1
  Switch3/1 -> Rudder/1
  Vel_in/1 -> Switch/1
  Switch/1 -> Throtlle/1
  Take-Off/4(Propeller) -> Switch/3
  Switch1/1 -> Profundor/1
  Take-Off/1(Elevators) -> Switch1/3
  Switch2/1 -> Aileron/1
  Saturation2/1 -> Switch2/1
  Saturation4/1 -> Switch1/1
  Saturation6/1 -> Switch3/1
  Gain1/1 -> Saturation6/1
  Yaw Attitude/1 -> Gain1/1
  Roll Attitude/1 -> Gain3/1
  Pitch Attitude/1 -> Gain2/1
  Gain2/1 -> Saturation4/1
  Gain3/1 -> Saturation2/1

== system SIL_swarm_Vasarhelyi/Cessna 4/High-Level/Gerador de Waypoints ==
  Xi : Inport
  Constant : Constant  Value=Radius_waypoint
  Constant1 : Constant  Value=Waypoints
  Constant2 : Constant  Value=N_Waypoints
  Constant3 : Constant  Value=p_swarm.r
  Display : Display
  Memory : Memory
  Next Waypoint : MATLAB Function  TreatAsAtomicUnit=on
  X Ref : Outport
  Y Ref : Outport  Port=2
  wires:
  Memory/1 -> Next Waypoint/6("Current_Waypoint ")
  Constant1/1 -> Next Waypoint/4(Waypoints)
  Xi/1 -> Next Waypoint/1(Xi)
  Constant3/1 -> Next Waypoint/3(p_swarm_r)
  Constant2/1 -> Next Waypoint/5(N_Waypoints)
  Next Waypoint/3(Current_Waypoint) -> Display/1, Memory/1
  Constant/1 -> Next Waypoint/2(R)
  Next Waypoint/1(X_ref) -> X Ref/1
  Next Waypoint/2(Y_ref) -> Y Ref/1

== system SIL_swarm_Vasarhelyi/Cessna 4/High-Level/Vasarhelyi Algorithm ==
  pos_i : Inport
  pqj : Inport  Port=2
  u_ref : Inport  Port=3
  Agents Number : Constant  Value=5
  Demux : Demux  Outputs=3
  Discrete Derivative : simulink/Discrete/Discrete Derivative  gainval=1.0  ICPrevScaledInput=0.0  OutMin=[]  OutMax=[]  OutDataType=fixdt(1, 16)  OutScaling=2^-10  DoSatur=off
  Discrete-Time Integrator : DiscreteIntegrator  SampleTime=-1  ICPrevOutput=DiscIntNeverNeededParam  ICPrevScaledInput=DiscIntNeverNeededParam
  Parameters : Subsystem
  Vasarhelyi Algorithm : MATLAB Function  TreatAsAtomicUnit=on
  dt : Constant  Value=0.01
  pos and vel of uavs : MATLAB Function  TreatAsAtomicUnit=on
  r_agent : Constant  Value=p_swarm.r_agent
  X : Outport
  Y : Outport  Port=2
  Z : Outport  Port=3
  Xi : Outport  Port=4
  wires:
  Agents Number/1 -> pos and vel of uavs/1(nb_agents)
  u_ref/1 -> Vasarhelyi Algorithm/4(u_ref)
  Vasarhelyi Algorithm/1(vel_command) -> Discrete-Time Integrator/1
  dt/1 -> Vasarhelyi Algorithm/5(dt)
  pqj/1 -> pos and vel of uavs/3(pqj)
  r_agent/1 -> Vasarhelyi Algorithm/6(r_agent)
  Discrete-Time Integrator/1 -> Demux/1
  pos and vel of uavs/1(pos) -> Discrete Derivative/1, Vasarhelyi Algorithm/2(pos), Xi/1
  Demux/2 -> Y/1
  pos_i/1 -> pos and vel of uavs/2(pos_i)
  Demux/1 -> X/1
  Demux/3 -> Z/1
  Discrete Derivative/1 -> Vasarhelyi Algorithm/3(vel)
  Parameters/1(p_swarm) -> Vasarhelyi Algorithm/1(p_swarm_par)

== system SIL_swarm_Vasarhelyi/Cessna 4/ROS Communication/Envio e Recepção de Dados do ROS ==
  note: ROS Receive
  Rudder : Inport
  Elevators : Inport  Port=2
  Flap : Inport  Port=3
  Aileron : Inport  Port=4
  Propeller : Inport  Port=5
  Blank Message : robotlib/Blank Message  messageClass=Message  entityType=aircraft_messages/Control_Surfaces  messageType=aircraft_messages/Control_Surfaces  SampleTime=-1  legacyBusStruct=off
  Bus Assignment1 : BusAssignment  AssignedSignals=Rudder,Elevators,RightFlap,RightAileron,Propeller
  Bus Selector1 : BusSelector  OutputSignals=Roll,Pitch,Yaw,PositionX,PositionY,PositionZ,Velocity
  Odometry : robotlib/Subscribe  topicSource=Select from ROS network  topic=/uav4/ground_truth/Odometry  messageType=aircraft_communication/Odom  SampleTime=-1  legacyBusStruct=off  messageQueueLength=1
  Publish : robotlib/Publish  topicSource=Select from ROS network  topic=/uav4/command  messageType=aircraft_messages/Control_Surfaces  legacyBusStruct=off  messageQueueLength=1
  Subscribe Odometry : Subsystem  TreatAsAtomicUnit=on
  Terminator1 : Terminator
  Terminator2 : Terminator
  Wifi Data : robotlib/Subscribe  topicSource=Select from ROS network  topic=/uav4/Communication  messageType=aircraft_communication/NetworkComm  SampleTime=-1  legacyBusStruct=off  messageQueueLength=1
  Pitch : Outport
  Yaw : Outport  Port=2
  Roll : Outport  Port=3
  ECEF X : Outport  Port=4
  ECEF Y : Outport  Port=5
  ECEF Z : Outport  Port=6
  Velocity : Outport  Port=7
  Xi : Outport  Port=8
  wires:
  Subscribe Odometry/5(ECEF Y) -> ECEF Y/1
  Subscribe Odometry/4(ECEF X) -> ECEF X/1
  Subscribe Odometry/2(Pitch) -> Pitch/1
  Subscribe Odometry/6(ECEF Z) -> ECEF Z/1
  Subscribe Odometry/8(Xi) -> Xi/1
  Subscribe Odometry/7(Velocity Out) -> Velocity/1
  Odometry/2 -> Bus Selector1/1
  Bus Selector1/4 -> Subscribe Odometry/4(ECEF_X)  "<PositionX>"
  Bus Selector1/5 -> Subscribe Odometry/5(ECEF_Y)  "<PositionY>"
  Bus Selector1/6 -> Subscribe Odometry/6(ECEF_Z)  "<PositionZ>"
  Wifi Data/2 -> Subscribe Odometry/8(Communication)
  Bus Selector1/7 -> Subscribe Odometry/7(Vel)  "<Velocity>"
  Bus Selector1/2 -> Subscribe Odometry/2(Pitch in)  "<Pitch>"
  Bus Selector1/1 -> Subscribe Odometry/1(Roll in)  "<Roll>"
  Bus Selector1/3 -> Subscribe Odometry/3(Yaw in)  "<Yaw>"
  Subscribe Odometry/3(Yaw) -> Yaw/1
  Subscribe Odometry/1(Roll) -> Roll/1
  Wifi Data/1 -> Terminator2/1
  Aileron/1 -> Bus Assignment1/5
  Blank Message/1 -> Bus Assignment1/1
  Flap/1 -> Bus Assignment1/4
  Elevators/1 -> Bus Assignment1/3
  Rudder/1 -> Bus Assignment1/2
  Bus Assignment1/1 -> Publish/1
  Propeller/1 -> Bus Assignment1/6
  Odometry/1 -> Terminator1/1

== system SIL_swarm_Vasarhelyi/Cessna 5/Attitude Control/Controle de Altitude ==
  Altitude Ref : Inport
  Altitude : Inport  Port=2
  Derivative1 : Derivative
  Kd : Gain  Gain=0.00162
  Kp : Gain  Gain=0.1
  Saturation : Saturate  UpperLimit=0.785398  LowerLimit=-0.785398
  Sum : Sum  Inputs=|+-
  Sum5 : Sum  Inputs=++|
  Pitch_ref : Outport
  altitude_error : Outport  Port=2
  wires:
  Saturation/1 -> Pitch_ref/1
  Altitude Ref/1 -> Sum/1
  Altitude/1 -> Sum/2
  Kp/1 -> Sum5/2
  Kd/1 -> Sum5/1
  Derivative1/1 -> Kd/1
  Sum5/1 -> Saturation/1
  Sum/1 -> Derivative1/1, Kp/1, altitude_error/1

== system SIL_swarm_Vasarhelyi/Cessna 5/Attitude Control/Controle de Velocidade ==
  Velocity Ref : Inport
  Velocity : Inport  Port=2
  K_prop : Gain  Gain=0.08
  PID Velocidade : Subsystem
  Propeller Ref : Constant  Value=0.7
  Saturation3 : Saturate  UpperLimit=0.8  LowerLimit=0.6
  Sum1 : Sum  Inputs=+|+
  Sum7 : Sum  Inputs=+|-
  Target Propeller : Scope
  Velocity Error : Scope
  Propeller Target : Outport
  velocity_error : Outport  Port=2
  wires:
  Velocity/1 -> Sum7/2
  Velocity Ref/1 -> Sum7/1
  PID Velocidade/1(ev) -> K_prop/1
  Saturation3/1 -> Target Propeller/1, Propeller Target/1
  Propeller Ref/1 -> Sum1/2
  K_prop/1 -> Sum1/1
  Sum1/1 -> Saturation3/1
  Sum7/1 -> PID Velocidade/1(e_vel), velocity_error/1, Velocity Error/1

== system SIL_swarm_Vasarhelyi/Cessna 5/Attitude Control/Servo ==
  Pitch Attitude : Inport
  Roll Attitude : Inport  Port=2
  Yaw Attitude : Inport  Port=3
  Vel_in : Inport  Port=4
  Altitude : Inport  Port=5
  Altitude Ref : Inport  Port=6
  Gain1 : Gain  Gain=-1
  Gain2 : Gain
  Gain3 : Gain
  GreaterThanOrEqual : RelationalOperator  OutDataTypeStr=boolean  RndMeth=Simplest
  Saturation2 : Saturate  UpperLimit=0.0523599  LowerLimit=-0.0523599
  Saturation4 : Saturate  UpperLimit=0.0523599  LowerLimit=-0.0523599
  Saturation6 : Saturate  UpperLimit=0.0872665  LowerLimit=-0.0872665
  Switch{,1..3} (4 alike) : Switch  Criteria=u2 ~= 0
  Take-Off : Subsystem
  Profundor : Outport
  Aileron : Outport  Port=2
  Rudder : Outport  Port=3
  Throtlle : Outport  Port=4
  wires:
  GreaterThanOrEqual/1 -> Switch3/2, Switch2/2, Switch1/2, Switch/2
  Altitude Ref/1 -> GreaterThanOrEqual/2
  Take-Off/3(Rudder) -> Switch3/3
  Take-Off/2(Aileron) -> Switch2/3
  Altitude/1 -> GreaterThanOrEqual/1
  Switch3/1 -> Rudder/1
  Vel_in/1 -> Switch/1
  Switch/1 -> Throtlle/1
  Take-Off/4(Propeller) -> Switch/3
  Switch1/1 -> Profundor/1
  Take-Off/1(Elevators) -> Switch1/3
  Switch2/1 -> Aileron/1
  Saturation2/1 -> Switch2/1
  Saturation4/1 -> Switch1/1
  Saturation6/1 -> Switch3/1
  Gain1/1 -> Saturation6/1
  Yaw Attitude/1 -> Gain1/1
  Roll Attitude/1 -> Gain3/1
  Pitch Attitude/1 -> Gain2/1
  Gain2/1 -> Saturation4/1
  Gain3/1 -> Saturation2/1

== system SIL_swarm_Vasarhelyi/Cessna 5/High-Level/Gerador de Waypoints ==
  Xi : Inport
  Constant : Constant  Value=Radius_waypoint
  Constant1 : Constant  Value=Waypoints
  Constant2 : Constant  Value=N_Waypoints
  Constant3 : Constant  Value=p_swarm.r
  Display : Display
  Memory : Memory
  Next Waypoint : MATLAB Function  TreatAsAtomicUnit=on
  X Ref : Outport
  Y Ref : Outport  Port=2
  wires:
  Memory/1 -> Next Waypoint/6("Current_Waypoint ")
  Constant1/1 -> Next Waypoint/4(Waypoints)
  Xi/1 -> Next Waypoint/1(Xi)
  Constant3/1 -> Next Waypoint/3(p_swarm_r)
  Constant2/1 -> Next Waypoint/5(N_Waypoints)
  Next Waypoint/3(Current_Waypoint) -> Display/1, Memory/1
  Constant/1 -> Next Waypoint/2(R)
  Next Waypoint/1(X_ref) -> X Ref/1
  Next Waypoint/2(Y_ref) -> Y Ref/1

== system SIL_swarm_Vasarhelyi/Cessna 5/High-Level/Vasarhelyi Algorithm ==
  pos_i : Inport
  pqj : Inport  Port=2
  u_ref : Inport  Port=3
  Agents Number : Constant  Value=5
  Demux : Demux  Outputs=3
  Discrete Derivative : simulink/Discrete/Discrete Derivative  gainval=1.0  ICPrevScaledInput=0.0  OutMin=[]  OutMax=[]  OutDataType=fixdt(1, 16)  OutScaling=2^-10  DoSatur=off
  Discrete-Time Integrator : DiscreteIntegrator  SampleTime=-1  ICPrevOutput=DiscIntNeverNeededParam  ICPrevScaledInput=DiscIntNeverNeededParam
  Parameters : Subsystem
  Vasarhelyi Algorithm : MATLAB Function  TreatAsAtomicUnit=on
  dt : Constant  Value=0.01
  pos and vel of uavs : MATLAB Function  TreatAsAtomicUnit=on
  r_agent : Constant  Value=p_swarm.r_agent
  X : Outport
  Y : Outport  Port=2
  Z : Outport  Port=3
  Xi : Outport  Port=4
  wires:
  Agents Number/1 -> pos and vel of uavs/1(nb_agents)
  u_ref/1 -> Vasarhelyi Algorithm/4(u_ref)
  Vasarhelyi Algorithm/1(vel_command) -> Discrete-Time Integrator/1
  dt/1 -> Vasarhelyi Algorithm/5(dt)
  pqj/1 -> pos and vel of uavs/3(pqj)
  r_agent/1 -> Vasarhelyi Algorithm/6(r_agent)
  Discrete-Time Integrator/1 -> Demux/1
  pos and vel of uavs/1(pos) -> Discrete Derivative/1, Vasarhelyi Algorithm/2(pos), Xi/1
  Demux/2 -> Y/1
  pos_i/1 -> pos and vel of uavs/2(pos_i)
  Demux/1 -> X/1
  Demux/3 -> Z/1
  Discrete Derivative/1 -> Vasarhelyi Algorithm/3(vel)
  Parameters/1(p_swarm) -> Vasarhelyi Algorithm/1(p_swarm_par)

== system SIL_swarm_Vasarhelyi/Cessna 5/ROS Communication/Envio e Recepção de Dados do ROS ==
  note: ROS Receive
  Rudder : Inport
  Elevators : Inport  Port=2
  Flap : Inport  Port=3
  Aileron : Inport  Port=4
  Propeller : Inport  Port=5
  Blank Message : robotlib/Blank Message  messageClass=Message  entityType=aircraft_messages/Control_Surfaces  messageType=aircraft_messages/Control_Surfaces  SampleTime=-1  legacyBusStruct=off
  Bus Assignment1 : BusAssignment  AssignedSignals=Rudder,Elevators,RightFlap,RightAileron,Propeller
  Bus Selector1 : BusSelector  OutputSignals=Roll,Pitch,Yaw,PositionX,PositionY,PositionZ,Velocity
  Odometry : robotlib/Subscribe  topicSource=Select from ROS network  topic=/uav5/ground_truth/Odometry  messageType=aircraft_communication/Odom  SampleTime=-1  legacyBusStruct=off  messageQueueLength=1
  Publish : robotlib/Publish  topicSource=Select from ROS network  topic=/uav5/command  messageType=aircraft_messages/Control_Surfaces  legacyBusStruct=off  messageQueueLength=1
  Subscribe Odometry : Subsystem  TreatAsAtomicUnit=on
  Terminator1 : Terminator
  Terminator2 : Terminator
  Wifi Data : robotlib/Subscribe  topicSource=Select from ROS network  topic=/uav5/Communication  messageType=aircraft_communication/NetworkComm  SampleTime=-1  legacyBusStruct=off  messageQueueLength=1
  Pitch : Outport
  Yaw : Outport  Port=2
  Roll : Outport  Port=3
  ECEF X : Outport  Port=4
  ECEF Y : Outport  Port=5
  ECEF Z : Outport  Port=6
  Velocity : Outport  Port=7
  Xi : Outport  Port=8
  wires:
  Subscribe Odometry/5(ECEF Y) -> ECEF Y/1
  Subscribe Odometry/4(ECEF X) -> ECEF X/1
  Subscribe Odometry/2(Pitch) -> Pitch/1
  Subscribe Odometry/6(ECEF Z) -> ECEF Z/1
  Subscribe Odometry/8(Xi) -> Xi/1
  Subscribe Odometry/7(Velocity Out) -> Velocity/1
  Odometry/2 -> Bus Selector1/1
  Bus Selector1/4 -> Subscribe Odometry/4(ECEF_X)  "<PositionX>"
  Bus Selector1/5 -> Subscribe Odometry/5(ECEF_Y)  "<PositionY>"
  Bus Selector1/6 -> Subscribe Odometry/6(ECEF_Z)  "<PositionZ>"
  Wifi Data/2 -> Subscribe Odometry/8(Communication)
  Bus Selector1/7 -> Subscribe Odometry/7(Vel)  "<Velocity>"
  Bus Selector1/2 -> Subscribe Odometry/2(Pitch in)  "<Pitch>"
  Bus Selector1/1 -> Subscribe Odometry/1(Roll in)  "<Roll>"
  Bus Selector1/3 -> Subscribe Odometry/3(Yaw in)  "<Yaw>"
  Subscribe Odometry/3(Yaw) -> Yaw/1
  Subscribe Odometry/1(Roll) -> Roll/1
  Wifi Data/1 -> Terminator2/1
  Aileron/1 -> Bus Assignment1/5
  Blank Message/1 -> Bus Assignment1/1
  Flap/1 -> Bus Assignment1/4
  Elevators/1 -> Bus Assignment1/3
  Rudder/1 -> Bus Assignment1/2
  Bus Assignment1/1 -> Publish/1
  Propeller/1 -> Bus Assignment1/6
  Odometry/1 -> Terminator1/1
